simulink model "known_case"  (R2021a)
settings: Solver=VariableStepAuto  StartTime=0.0  StopTime=20.0  RelTol=1e-3
libraries: simulink x1
settings Model: SimulationMode=accelerator  Creator=tejal  LastModifiedBy=dhruv

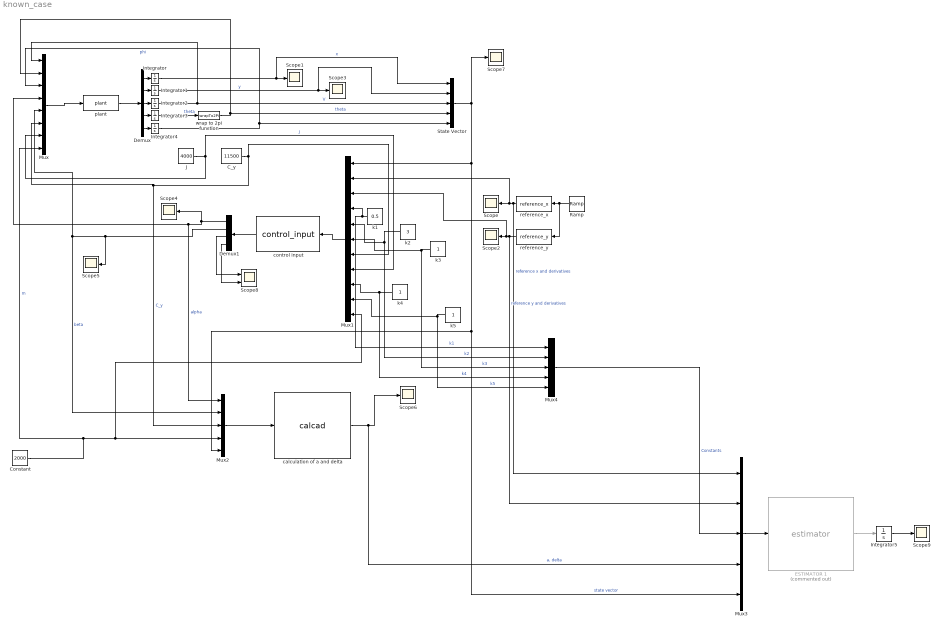
== system known_case ==
  C_y : Constant  Value=11500
  Constant : Constant  Value=2000
  Demux : Demux  Outputs=5
  Demux1 : Demux
  ESTIMATOR 1 : MATLABFcn  Commented=on  MATLABFcn=estimator  OutputDimensions=4
  Integrator : Integrator  InitialCondition=0.0005
  Integrator1 : Integrator  InitialCondition=0.00005
  Integrator2 : Integrator  InitialCondition=1  UpperSaturationLimit=100  LowerSaturationLimit=-10
  Integrator3 : Integrator  InitialCondition=0.7
  Integrator4 : Integrator  UpperSaturationLimit=100  LowerSaturationLimit=-100
  Integrator5 : Integrator  InitialCondition=[5.75;0.5;2.875;11.5]
  J : Constant  Value=4000
  Mux : Mux  Inputs=8
  Mux1 : Mux  Inputs=11
  Mux2 : Mux  Inputs=5
  Mux3 : Mux  Inputs=5
  Mux4 : Mux  Inputs=5
  Ramp : simulink/Sources/Ramp  slope=1  start=0  InitialOutput=0
  Scope{,1..7,9} (9 alike) : Scope
  Scope8 : Scope  NumInputPorts=2
  State Vector : Mux  Inputs=5
  calculation of a and delta : MATLABFcn  MATLABFcn=calcad  OutputDimensions=2
  control input : MATLABFcn  MATLABFcn=control_input  OutputDimensions=4
  k1 : Constant  Value=0.5
  k2 : Constant  Value=3
  k3 : Constant
  k4 : Constant
  k5 : Constant
  plant : MATLABFcn  MATLABFcn=plant  OutputDimensions=5
  reference_x : MATLABFcn  MATLABFcn=reference_x  OutputDimensions=4
  reference_y : MATLABFcn  MATLABFcn=reference_y  OutputDimensions=4
  wrap to 2pi function : MATLABFcn  MATLABFcn=wrapTo2Pi
  wires:
  Ramp/1 -> reference_y/1, reference_x/1
  Mux/1 -> plant/1
  plant/1 -> Demux/1
  Demux/1 -> Integrator/1
  Demux/5 -> Integrator4/1
  Demux/4 -> Integrator3/1
  Demux/3 -> Integrator2/1
  Demux/2 -> Integrator1/1
  Integrator/1 -> State Vector/1, Scope1/1  "x"
  Integrator1/1 -> State Vector/2, Scope3/1  "y"
  Integrator2/1 -> Mux/1, State Vector/3  "V"
  Integrator3/1 -> wrap to 2pi function/1  "theta"
  Integrator4/1 -> State Vector/5, Mux/3  "phi"
  J/1 -> Mux/7, Mux1/8  "J"
  control input/1 -> Demux1/1
  Mux1/1 -> control input/1
  wrap to 2pi function/1 -> State Vector/4, Mux/2  "theta"
  Demux1/3 -> Scope8/1
  Demux1/4 -> Scope8/2
  Mux2/1 -> calculation of a and delta/1
  C_y/1 -> Mux2/3, Mux/6, Mux1/7  "C_y"
  Demux1/2 -> Scope5/1, Mux2/2, Mux/5  "beta"
  Demux1/1 -> Mux2/1, Mux/4, Scope4/1  "alpha"
  Constant/1 -> Mux/8, Mux1/11, Mux2/4  "m"
  Mux4/1 -> Mux3/3  "Constants"
  State Vector/1 -> Mux3/5, Mux2/5, Mux1/1, Scope7/1  "state vector"
  Mux3/1 -> ESTIMATOR 1/1
  ESTIMATOR 1/1 -> Integrator5/1
  reference_y/1 -> Mux3/2, Mux1/3, Scope2/1  "reference y and derivatives"
  calculation of a and delta/1 -> Mux3/4, Scope6/1  "a, delta"
  Integrator5/1 -> Scope9/1
  reference_x/1 -> Mux3/1, Mux1/2, Scope/1  "reference x and derivatives"
  k4/1 -> Mux1/9, Mux4/4  "k4"
  k5/1 -> Mux1/10, Mux4/5  "k5"
  k2/1 -> Mux4/2, Mux1/5  "k2"
  k1/1 -> Mux4/1, Mux1/4  "k1"
  k3/1 -> Mux1/6, Mux4/3  "k3"
